simulink model "model15062023"  (R2021a)
settings: Solver=VariableStepAuto  StartTime=0.0  StopTime=10  FixedStep=1e-3  RelTol=1e-5
values from neighbouring files (symbols this model uses):
  I_max = 3*I_nom    (= 57.3875996726)    [LIM_parameters.m]
  I_min = 0.1*I_nom    (= 1.91291998909)    [LIM_parameters.m]
  I_nom = psi_ref/L_M_hat    (= 19.1291998909)    [LIM_parameters.m]
  ki_c = alpha_c*(R_hat+Ra )    [LIM_parameters.m]
  ki_s = alpha_s^2*m_hat/ psi_ref    [LIM_parameters.m]
  kp_c = alpha_c*L_sigma_hat    [LIM_parameters.m]
  kp_s = alpha_s*m_hat/ psi_ref    [LIM_parameters.m]
  L = 1    [LIM_parameters.m]
  L_alpha = (Ls+Lm)*(Lr+Lm) -Lm^2    (= 0.00742144)    [LIM_parameters.m]
  L_sigma_hat = L_sigma    (= 0.0268)    [LIM_parameters.m]
  Lm = 0.0416    [LIM_parameters.m]    (also in LIMvariables.m = 0.0376)
  Lr = 0.0416    [LIM_parameters.m]
  Ls = 0.0684    [LIM_parameters.m]
  m = 10    [LIM_parameters.m]    (also in LIMvariables.m)
  p = 4    [LIM_parameters.m]
  psi_ref = 1*250/(100*pi )    (= 0.795774715459)    [LIM_parameters.m]
  R_R_hat = Rr    (= 0.976)    [LIM_parameters.m]
  Ra = alpha_c*L_sigma_hat - R_hat    [LIM_parameters.m]
  Rr = 0.976    [LIM_parameters.m]
  Rs = 1.298    [LIM_parameters.m]
  tau = L/p    (= 0.25)    [LIM_parameters.m]    (also in LIMvariables.m = 0.066)
  V_sat = 415*sqrt(2/3)    [LIM_parameters.m]
  Vbase = 250    [LIM_parameters.m]
  wbase_fw = 50*2*pi    (= 314.159265359)    [LIM_parameters.m]
  zeta = (L_sigma_hat+L_M_hat)/L_sigma_hat    (= 2.55223880597)    [LIM_parameters.m]
libraries: simulink x5
settings Model: Creator=r.pitarque  LastModifiedBy=Asus

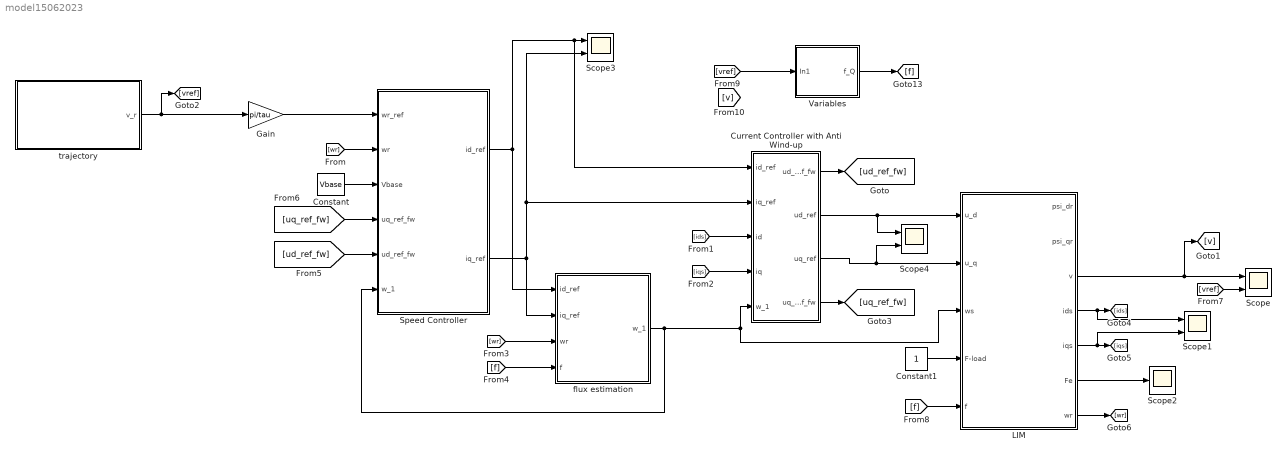
== system model15062023 ==
  Constant : Constant  Value=Vbase
  Constant1 : Constant
  Current Controller with Anti Wind-up : Subsystem
  Gain : Gain  Gain=pi/tau
  LIM : Subsystem
  Scope{,1,3..4} (4 alike) : Scope  NumInputPorts=2
  Scope2 : Scope
  Speed Controller : Subsystem
  Variables : Subsystem
  flux estimation : Subsystem
  trajectory : Subsystem
  wires:
  Current Controller with Anti Wind-up/1(ud_ref_fw) -> [ud_ref_fw]
  Current Controller with Anti Wind-up/2(ud_ref) -> Scope4/1, LIM/1(u_d)
  Current Controller with Anti Wind-up/3(uq_ref) -> Scope4/2, LIM/2(u_q)
  Current Controller with Anti Wind-up/4(uq_ref_fw) -> [uq_ref_fw]
  Speed Controller/1(id_ref) -> flux estimation/1(id_ref), Current Controller with Anti Wind-up/1(id_ref), Scope3/1
  LIM/4(ids) -> Scope1/1, [ids]
  LIM/5(iqs) -> Scope1/2, [iqs]
  LIM/7(wr) -> [wr]
  [wr] -> Speed Controller/2(wr)
  [ids] -> Current Controller with Anti Wind-up/3(id)
  [iqs] -> Current Controller with Anti Wind-up/4(iq)
  flux estimation/1(w_1) -> Speed Controller/6(w_1), Current Controller with Anti Wind-up/5(w_1), LIM/3(ws)
  [wr] -> flux estimation/3(wr)
  [f] -> flux estimation/4(f)
  Constant/1 -> Speed Controller/3(Vbase)
  [ud_ref_fw] -> Speed Controller/5(ud_ref_fw)
  [uq_ref_fw] -> Speed Controller/4(uq_ref_fw)
  trajectory/1(v_r) -> Gain/1, [vref]
  Gain/1 -> Speed Controller/1(wr_ref)
  LIM/3(v) -> [v], Scope/1
  [vref] -> Scope/2
  Variables/1(f_Q) -> [f]
  [f] -> LIM/5(f)
  LIM/6(Fe) -> Scope2/1
  Constant1/1 -> LIM/4(F-load)
  Speed Controller/2(iq_ref) -> flux estimation/2(iq_ref), Current Controller with Anti Wind-up/2(iq_ref), Scope3/2
  [vref] -> Variables/1(In1)

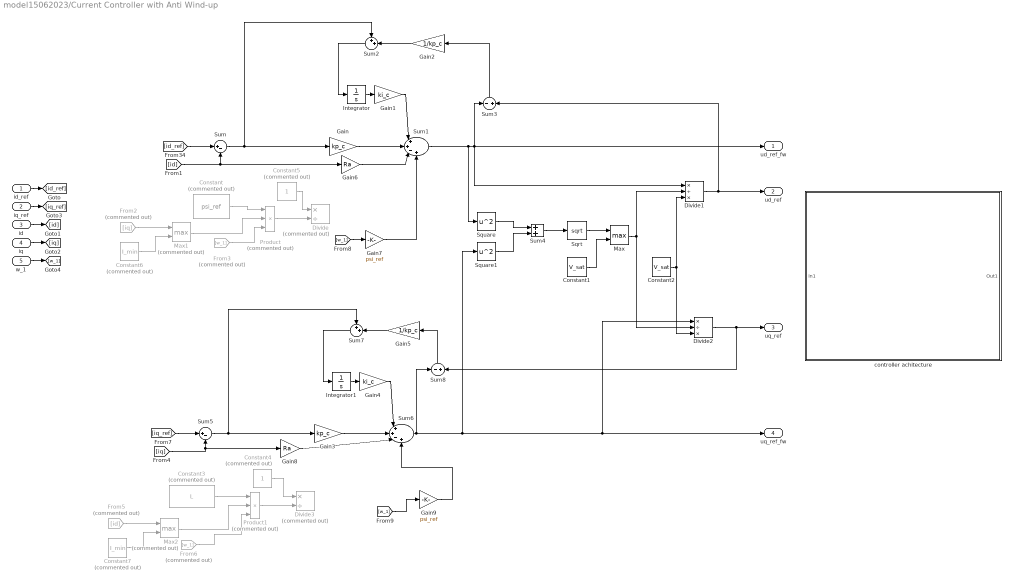
== system model15062023/Current Controller with Anti Wind-up ==
  id_ref : Inport
  iq_ref : Inport  Port=2
  id : Inport  Port=3
  iq : Inport  Port=4
  w_1 : Inport  Port=5
  Constant : Constant  Commented=on  Value=psi_ref
  Constant1 : Constant  Value=V_sat
  Constant2 : Constant  Value=V_sat
  Constant3 : Constant  Commented=on  Value=L
  Constant4 : Constant  Commented=on
  Constant5 : Constant  Commented=on
  Constant6 : Constant  Commented=on  Value=I_min
  Constant7 : Constant  Commented=on  Value=I_min
  Divide : Product  Commented=on  Inputs=*/
  Divide1 : Product  Inputs=*/*
  Divide2 : Product  Inputs=*/*
  Divide3 : Product  Commented=on  Inputs=*/
  From2 : From  Commented=on  GotoTag=iq
  From3 : From  Commented=on  GotoTag=w_1
  From5 : From  Commented=on  GotoTag=id
  From6 : From  Commented=on  GotoTag=w_1
  Gain : Gain  Gain=kp_c
  Gain1 : Gain  Gain=ki_c
  Gain2 : Gain  Gain=1/kp_c
  Gain3 : Gain  Gain=kp_c
  Gain4 : Gain  Gain=ki_c
  Gain5 : Gain  Gain=1/kp_c
  Gain6 : Gain  Gain=Ra
  Gain7 : Gain  Gain=psi_ref
  Gain8 : Gain  Gain=Ra
  Gain9 : Gain  Gain=psi_ref
  Integrator : Integrator
  Integrator1 : Integrator
  Max : MinMax  Function=max  Inputs=2
  Max1 : MinMax  Commented=on  Function=max  Inputs=2
  Max2 : MinMax  Commented=on  Function=max  Inputs=2
  Product : Product  Commented=on  Inputs=3
  Product1 : Product  Commented=on  Inputs=3
  Sqrt : Sqrt  SaturateOnIntegerOverflow=on
  Square : Math  Operator=square  SaturateOnIntegerOverflow=on
  Square1 : Math  Operator=square  SaturateOnIntegerOverflow=on
  Sum : Sum  Inputs=|+-
  Sum1 : Sum  Inputs=|++-+
  Sum2 : Sum  Inputs=++|
  Sum3 : Sum  Inputs=-+
  Sum4 : Sum
  Sum5 : Sum  Inputs=|+-
  Sum6 : Sum  Inputs=|++-+
  Sum7 : Sum  Inputs=++|
  Sum8 : Sum  Inputs=-+
  controller achitecture : Subsystem
      mask Display: image('C:\Users\Asus\Desktop\cc.png'); % Use "Edit Image" on toolstrip to change.
  ud_ref_fw : Outport
  ud_ref : Outport  Port=2
  uq_ref : Outport  Port=3
  uq_ref_fw : Outport  Port=4
  wires:
  Square/1 -> Sum4/1
  Constant1/1 -> Max/2
  Sum6/1 -> Sum8/1, uq_ref_fw/1, Divide2/1, Square1/1
  Max/1 -> Divide2/2, Divide1/2
  Sum1/1 -> ud_ref_fw/1, Sum3/1, Divide1/1, Square/1
  Constant3/1 -> Product1/1
  Square1/1 -> Sum4/2
  Constant2/1 -> Divide1/3, Divide2/3
  Gain1/1 -> Sum1/1
  Divide2/1 -> uq_ref/1, Sum8/2
  Sqrt/1 -> Max/1
  Sum/1 -> Gain/1, Sum2/1
  Sum4/1 -> Sqrt/1
  Product/1 -> Divide/2
  Gain2/1 -> Sum2/2
  Divide1/1 -> ud_ref/1, Sum3/2
  Integrator/1 -> Gain1/1
  Sum5/1 -> Gain3/1, Sum7/1
  Constant/1 -> Product/1
  Gain/1 -> Sum1/2
  Integrator1/1 -> Gain4/1
  Gain4/1 -> Sum6/1
  Sum3/1 -> Gain2/1
  Sum7/1 -> Integrator1/1
  Gain3/1 -> Sum6/2
  Product1/1 -> Divide3/2
  Sum8/1 -> Gain5/1
  Sum2/1 -> Integrator/1
  [id_ref] -> Sum/1
  [id] -> Gain6/1, Sum/2
  From6/1 -> Product1/3
  [iq_ref] -> Sum5/1
  [iq] -> Gain8/1, Sum5/2
  From2/1 -> Max1/1
  From3/1 -> Product/3
  id/1 -> [id]
  iq/1 -> [iq]
  w_1/1 -> [w_1]
  iq_ref/1 -> [iq_ref]
  id_ref/1 -> [id_ref]
  Gain5/1 -> Sum7/2
  Constant4/1 -> Divide3/1
  Constant5/1 -> Divide/1
  Constant6/1 -> Max1/2
  Max1/1 -> Product/2
  Constant7/1 -> Max2/2
  From5/1 -> Max2/1
  Max2/1 -> Product1/2
  Gain6/1 -> Sum1/3
  [w_1] -> Gain7/1
  Gain7/1 -> Sum1/4
  Gain8/1 -> Sum6/3
  [w_1] -> Gain9/1
  Gain9/1 -> Sum6/4

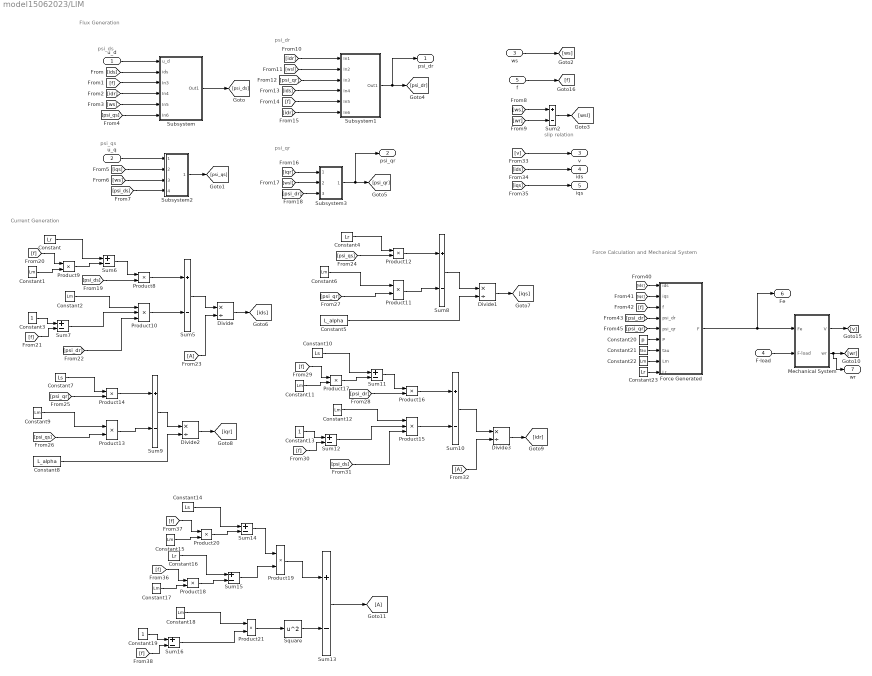
== system model15062023/LIM ==
  note: Force Calculation and Mechanical System
  note: Current Generation
  note: Flux Generation
  note: psi_qr
  note: psi_dr
  note: psi_qs
  note: psi_ds
  note: slip relation
  u_d : Inport
  u_q : Inport  Port=2
  ws : Inport  Port=3
  F-load : Inport  Port=4
  f : Inport  Port=5
  Constant{,4,16,23} (4 alike) : Constant  Value=Lr
  Constant{1..2,6,9,11..12,15,17..18,22} (10 alike) : Constant  Value=Lm
  Constant10 : Constant  Value=Ls
  Constant13 : Constant
  Constant14 : Constant  Value=Ls
  Constant19 : Constant
  Constant20 : Constant  Value=p
  Constant21 : Constant  Value=tau
  Constant3 : Constant
  Constant5 : Constant  Value=L_alpha
  Constant7 : Constant  Value=Ls
  Constant8 : Constant  Value=L_alpha
  Divide{,1..3} (4 alike) : Product  Inputs=*/
  Force Generated : MATLAB Function  TreatAsAtomicUnit=on
  Mechanical System : Subsystem
  Product10 : Product  Inputs=3
  Product{8..9,11..14,16..21} (12 alike) : Product
  Product15 : Product  Inputs=3
  Square : Math  Operator=square  SaturateOnIntegerOverflow=on
  Subsystem : Subsystem
  Subsystem1 : Subsystem
  Subsystem2 : Subsystem
  Subsystem3 : Subsystem
  Sum{2,5..16} (13 alike) : Sum  Inputs=+-
  psi_dr : Outport
  psi_qr : Outport  Port=2
  v : Outport  Port=3
  ids : Outport  Port=4
  iqs : Outport  Port=5
  Fe : Outport  Port=6
  wr : Outport  Port=7
  wires:
  [f] -> Sum16/2
  [psi_qs] -> Product12/2
  Constant3/1 -> Sum7/1
  Constant16/1 -> Sum15/1
  [v] -> v/1
  Divide1/1 -> [iqs]
  Constant19/1 -> Sum16/1
  [f] -> Sum7/2
  [ws] -> Sum2/1
  Sum5/1 -> Divide/1
  Constant12/1 -> Product15/1
  Sum6/1 -> Product8/1
  [psi_dr] -> Subsystem3/3(In3)
  Divide/1 -> [ids]
  [psi_qr] -> Force Generated/5(psi_qr)
  [A] -> Divide/2
  Sum13/1 -> [A]
  [f] -> Product17/1
  Product10/1 -> Sum5/2
  Force Generated/1(F) -> Fe/1, Mechanical System/1(Fe)
  [psi_ds] -> Product15/3
  [psi_qr] -> Product11/2
  Constant8/1 -> Divide2/2
  Divide2/1 -> [iqr]
  Sum7/1 -> Product10/2
  Constant14/1 -> Sum14/1
  F-load/1 -> Mechanical System/2(F-load)
  [iqs] -> iqs/1
  Constant9/1 -> Product13/1
  Sum2/1 -> [wsl]
  Sum9/1 -> Divide2/1
  [f] -> Product9/1
  Sum8/1 -> Divide1/1
  Product13/1 -> Sum9/2
  Constant1/1 -> Product9/2
  [psi_qr] -> Product14/2
  Constant7/1 -> Product14/1
  Square/1 -> Sum13/2
  [wsl] -> Subsystem1/2(In2)
  Product14/1 -> Sum9/1
  [idr] -> Subsystem1/1(In1)
  [ids] -> Force Generated/1(ids)
  [psi_qs] -> Product13/2
  [idr] -> Subsystem1/6(In6)
  [psi_qr] -> Subsystem1/3(In3)
  Product12/1 -> Sum8/1
  Mechanical System/2(wr) -> wr/1, [wr]
  Subsystem1/1(Out1) -> psi_dr/1, [psi_dr]
  [f] -> Product20/1
  Product21/1 -> Square/1
  Product11/1 -> Sum8/2
  Sum15/1 -> Product19/2
  Product9/1 -> Sum6/2
  Subsystem/1(Out1) -> [psi_ds]
  Subsystem3/1(Out1) -> psi_qr/1, [psi_qr]
  Constant2/1 -> Product10/1
  [f] -> Subsystem1/5(In5)
  ws/1 -> [ws]
  [wr] -> Sum2/2
  [psi_dr] -> Product10/3
  [psi_dr] -> Force Generated/4(psi_dr)
  Constant18/1 -> Product21/1
  [ws] -> Subsystem2/3(In3)
  Constant4/1 -> Product12/1
  Constant/1 -> Sum6/1
  Constant6/1 -> Product11/1
  Constant21/1 -> Force Generated/7(tau)
  Product8/1 -> Sum5/1
  [f] -> Product18/1
  Constant17/1 -> Product18/2
  Product18/1 -> Sum15/2
  [psi_ds] -> Product8/2
  Constant5/1 -> Divide1/2
  Sum16/1 -> Product21/2
  [psi_dr] -> Product16/2
  Product16/1 -> Sum10/1
  Sum12/1 -> Product15/2
  Constant11/1 -> Product17/2
  [f] -> Sum12/2
  Constant10/1 -> Sum11/1
  Product17/1 -> Sum11/2
  Product15/1 -> Sum10/2
  [A] -> Divide3/2
  Constant23/1 -> Force Generated/9(Lr)
  Divide3/1 -> [idr]
  Constant13/1 -> Sum12/1
  Sum11/1 -> Product16/1
  Sum10/1 -> Divide3/1
  [ids] -> ids/1
  Product20/1 -> Sum14/2
  Constant15/1 -> Product20/2
  Sum14/1 -> Product19/1
  Product19/1 -> Sum13/1
  Mechanical System/1(V) -> [v]
  [f] -> Force Generated/3(f)
  Constant20/1 -> Force Generated/6(P)
  [ws] -> Subsystem/5(In5)
  [psi_qs] -> Subsystem/6(In6)
  u_d/1 -> Subsystem/1(u_d)
  [idr] -> Subsystem/4(In4)
  [f] -> Subsystem/3(In3)
  [ids] -> Subsystem/2(ids)
  [iqs] -> Force Generated/2(iqs)
  [ids] -> Subsystem1/4(In4)
  [iqr] -> Subsystem3/1(In1)
  [wsl] -> Subsystem3/2(In2)
  [psi_ds] -> Subsystem2/4(In4)
  Subsystem2/1(Out1) -> [psi_qs]
  [iqs] -> Subsystem2/2(In2)
  u_q/1 -> Subsystem2/1(In1)
  Constant22/1 -> Force Generated/8(Lm)
  f/1 -> [f]

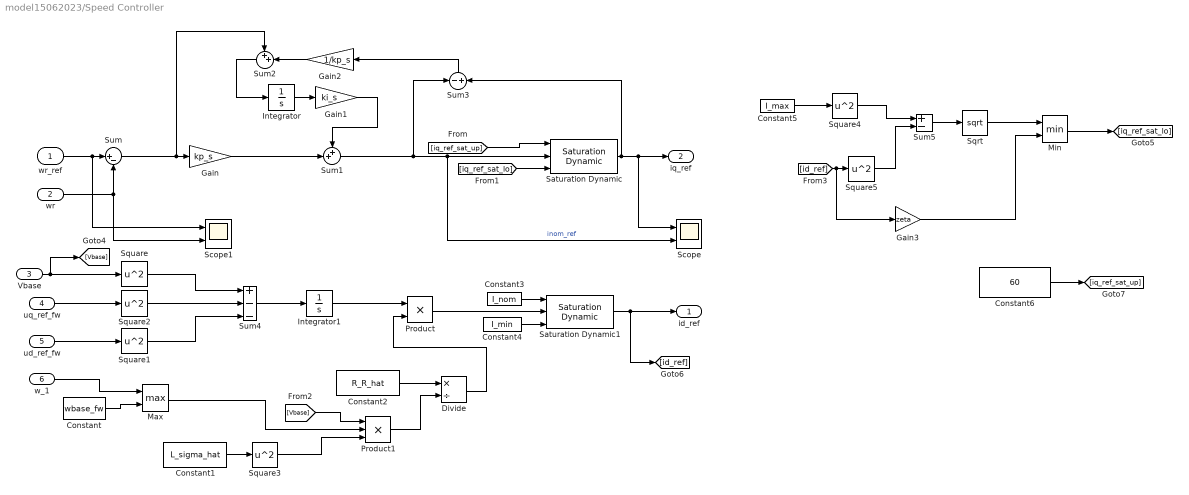
== system model15062023/Speed Controller ==
  wr_ref : Inport
  wr : Inport  Port=2
  Vbase : Inport  Port=3
  uq_ref_fw : Inport  Port=4
  ud_ref_fw : Inport  Port=5
  w_1 : Inport  Port=6
  Constant : Constant  Value=wbase_fw
  Constant1 : Constant  Value=L_sigma_hat
  Constant2 : Constant  Value=R_R_hat
  Constant3 : Constant  Value=I_nom
  Constant4 : Constant  Value=I_min
  Constant5 : Constant  Value=I_max
  Constant6 : Constant  Value=60
  Divide : Product  Inputs=*/
  Gain : Gain  Gain=kp_s
  Gain1 : Gain  Gain=ki_s
  Gain2 : Gain  Gain=1/kp_s
  Gain3 : Gain  Gain=zeta
  Integrator : Integrator
  Integrator1 : Integrator
  Max : MinMax  Function=max  Inputs=2
  Min : MinMax  Inputs=2
  Product : Product
  Product1 : Product  Inputs=3
  Saturation Dynamic : simulink/Discontinuities/Saturation Dynamic  OutMin=[]  OutMax=[]  OutDataTypeStr=Inherit: Same as second input  OutDataType=fixdt(1, 16)  OutScaling=2^-10  DoSatur=off
  Saturation Dynamic1 : simulink/Discontinuities/Saturation Dynamic  OutMin=[]  OutMax=[]  OutDataTypeStr=Inherit: Same as second input  OutDataType=fixdt(1, 16)  OutScaling=2^-10  DoSatur=off
  Scope : Scope  NumInputPorts=2
  Scope1 : Scope  NumInputPorts=2
  Sqrt : Sqrt  SaturateOnIntegerOverflow=on
  Square{,1..5} (6 alike) : Math  Operator=square  SaturateOnIntegerOverflow=on
  Sum : Sum  Inputs=|+-
  Sum1 : Sum  Inputs=++|
  Sum2 : Sum  Inputs=++|
  Sum3 : Sum  Inputs=-+
  Sum4 : Sum  Inputs=+--
  Sum5 : Sum  Inputs=+-
  id_ref : Outport
  iq_ref : Outport  Port=2
  wires:
  Constant2/1 -> Divide/1
  Integrator1/1 -> Product/1
  Gain2/1 -> Sum2/2
  Square1/1 -> Sum4/3
  Min/1 -> [iq_ref_sat_lo]
  Constant5/1 -> Square4/1
  Vbase/1 -> [Vbase], Square/1
  Constant4/1 -> Saturation Dynamic1/3
  Gain3/1 -> Min/2
  Sum/1 -> Sum2/1, Gain/1
  Product1/1 -> Divide/2
  Constant3/1 -> Saturation Dynamic1/1
  [Vbase] -> Product1/1
  Max/1 -> Product1/2
  Square5/1 -> Sum5/2
  Saturation Dynamic1/1 -> id_ref/1, [id_ref]
  Constant/1 -> Max/2
  [iq_ref_sat_lo] -> Saturation Dynamic/3
  [id_ref] -> Gain3/1, Square5/1
  Gain/1 -> Sum1/2
  uq_ref_fw/1 -> Square2/1
  Sum5/1 -> Sqrt/1
  Constant1/1 -> Square3/1
  Sum4/1 -> Integrator1/1
  Sum3/1 -> Gain2/1
  Product/1 -> Saturation Dynamic1/2
  Square2/1 -> Sum4/2
  [iq_ref_sat_up] -> Saturation Dynamic/1
  ud_ref_fw/1 -> Square1/1
  Divide/1 -> Product/2
  Sqrt/1 -> Min/1
  Square4/1 -> Sum5/1
  Sum2/1 -> Integrator/1
  wr/1 -> Scope1/2, Sum/2
  Square/1 -> Sum4/1
  Sum1/1 -> Scope/2, Saturation Dynamic/2, Sum3/1  "inom_ref"
  w_1/1 -> Max/1
  Constant6/1 -> [iq_ref_sat_up]
  Integrator/1 -> Gain1/1
  Square3/1 -> Product1/3
  Saturation Dynamic/1 -> Scope/1, iq_ref/1, Sum3/2
  Gain1/1 -> Sum1/1
  wr_ref/1 -> Scope1/1, Sum/1

== system model15062023/Variables ==
  In1 : Inport
  Gain : Gain  Gain=L*Rr/Lr
  Subsystem5 : Subsystem  Commented=on
  f(Q) : MATLAB Function  TreatAsAtomicUnit=on
  f_Q : Outport
  wires:
  Gain/1 -> f(Q)/1(u)  "Q"
  f(Q)/1(y) -> f_Q/1, Subsystem5/1(f_q)  "F_Q"
  Subsystem5/1(Lsigma) -> ?
  In1/1 -> Gain/1

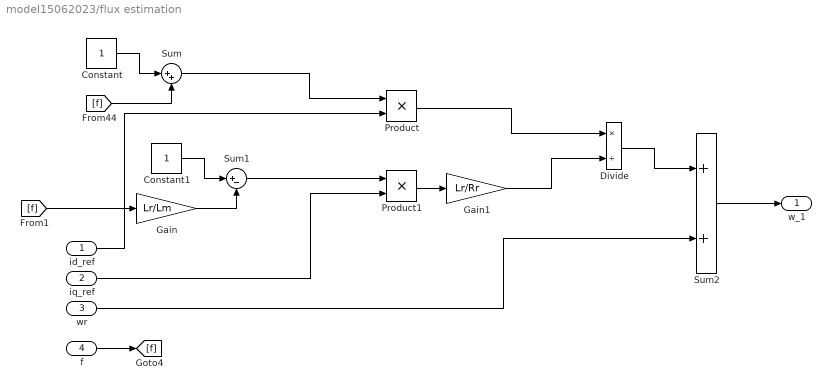
== system model15062023/flux estimation ==
  id_ref : Inport
  iq_ref : Inport  Port=2
  wr : Inport  Port=3
  f : Inport  Port=4
  Constant : Constant
  Constant1 : Constant
  Divide : Product  Inputs=*/
  Gain : Gain  Gain=Lr/Lm
  Gain1 : Gain  Gain=Lr/Rr
  Product : Product
  Product1 : Product
  Sum : Sum  Inputs=|++
  Sum1 : Sum  Inputs=|+-
  Sum2 : Sum
  w_1 : Outport
  wires:
  Sum1/1 -> Product1/1
  Divide/1 -> Sum2/1
  wr/1 -> Sum2/2
  Product/1 -> Divide/1
  Constant/1 -> Sum/1
  Gain/1 -> Sum1/2
  id_ref/1 -> Product/2
  Gain1/1 -> Divide/2
  [f] -> Sum/2
  Product1/1 -> Gain1/1
  Sum/1 -> Product/1
  Constant1/1 -> Sum1/1
  [f] -> Gain/1
  iq_ref/1 -> Product1/2
  f/1 -> [f]
  Sum2/1 -> w_1/1

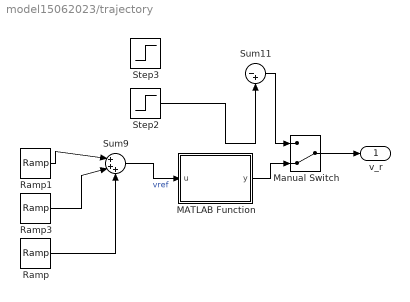
== system model15062023/trajectory ==
  MATLAB Function : MATLAB Function  TreatAsAtomicUnit=on
  Manual Switch : ManualSwitch  CurrentSetting=0
  Ramp : simulink/Sources/Ramp  slope=-6.5  start=5.28  InitialOutput=0
  Ramp1 : simulink/Sources/Ramp  slope=4.12  start=0  InitialOutput=0.1
  Ramp3 : simulink/Sources/Ramp  slope=-4.12  start=5.28  InitialOutput=0.1
  Step2 : Step  Time=0  Before=0.1  SampleTime=0
  Step3 : Step  Time=4  Before=20  After=0.1  SampleTime=0
  Sum11 : Sum  Inputs=|-+
  Sum9 : Sum  Inputs=|+++
  v_r : Outport
  wires:
  MATLAB Function/1(y) -> Manual Switch/2
  Sum11/1 -> Manual Switch/1
  Ramp3/1 -> Sum9/2
  Step2/1 -> Sum11/2
  Ramp/1 -> Sum9/3
  Ramp1/1 -> Sum9/1
  Manual Switch/1 -> v_r/1
  Sum9/1 -> MATLAB Function/1(u)  "vref"

== system model15062023/Current Controller with Anti Wind-up/controller achitecture ==
  In1 : Inport
  Out1 : Outport
  wires:
  In1/1 -> Out1/1

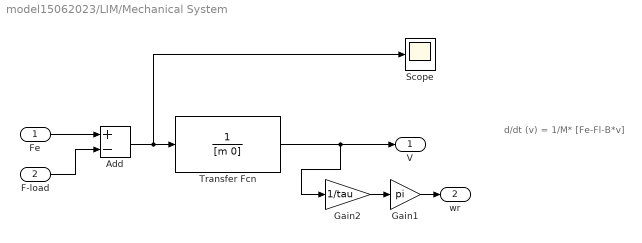
== system model15062023/LIM/Mechanical System ==
  note: d/dt (v) = 1/M* [Fe-Fl-B*v]
  Fe : Inport
  F-load : Inport  Port=2
  Add : Sum  Inputs=+-
  Gain1 : Gain  Gain=pi
  Gain2 : Gain  Gain=1/tau
  Scope : Scope
  Transfer Fcn : TransferFcn  Denominator=[m 0]
  V : Outport
  wr : Outport  Port=2
  wires:
  Fe/1 -> Add/1
  F-load/1 -> Add/2
  Add/1 -> Scope/1, Transfer Fcn/1
  Gain2/1 -> Gain1/1
  Gain1/1 -> wr/1
  Transfer Fcn/1 -> Gain2/1, V/1

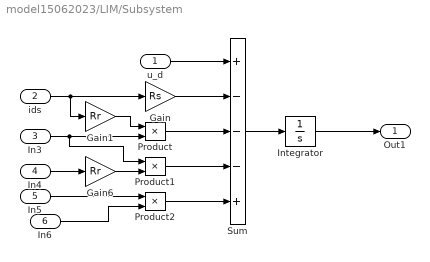
== system model15062023/LIM/Subsystem ==
  u_d : Inport
  ids : Inport  Port=2
  In3 : Inport  Port=3
  In4 : Inport  Port=4
  In5 : Inport  Port=5
  In6 : Inport  Port=6
  Gain : Gain  Gain=Rs
  Gain1 : Gain  Gain=Rr
  Gain6 : Gain  Gain=Rr
  Integrator : Integrator
  Product : Product
  Product1 : Product
  Product2 : Product
  Sum : Sum  Inputs=+---+
  Out1 : Outport
  wires:
  Gain1/1 -> Product/1
  Product/1 -> Sum/3
  ids/1 -> Gain1/1, Gain/1
  Product2/1 -> Sum/5
  Gain/1 -> Sum/2
  In3/1 -> Product1/1, Product/2
  u_d/1 -> Sum/1
  Product1/1 -> Sum/4
  Sum/1 -> Integrator/1
  Gain6/1 -> Product1/2
  In5/1 -> Product2/1
  In6/1 -> Product2/2
  In4/1 -> Gain6/1
  Integrator/1 -> Out1/1

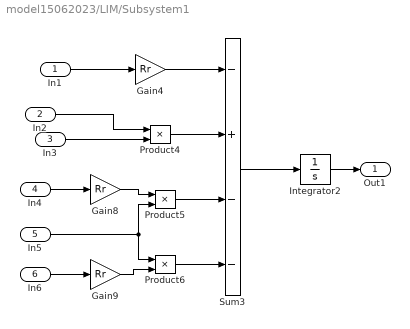
== system model15062023/LIM/Subsystem1 ==
  In1 : Inport
  In2 : Inport  Port=2
  In3 : Inport  Port=3
  In4 : Inport  Port=4
  In5 : Inport  Port=5
  In6 : Inport  Port=6
  Gain4 : Gain  Gain=Rr
  Gain8 : Gain  Gain=Rr
  Gain9 : Gain  Gain=Rr
  Integrator2 : Integrator
  Product4 : Product
  Product5 : Product
  Product6 : Product
  Sum3 : Sum  Inputs=-+--
  Out1 : Outport
  wires:
  Gain9/1 -> Product6/2
  Product4/1 -> Sum3/2
  Product6/1 -> Sum3/4
  Integrator2/1 -> Out1/1
  Gain8/1 -> Product5/1
  In5/1 -> Product6/1, Product5/2
  Sum3/1 -> Integrator2/1
  Product5/1 -> Sum3/3
  Gain4/1 -> Sum3/1
  In1/1 -> Gain4/1
  In3/1 -> Product4/2
  In2/1 -> Product4/1
  In4/1 -> Gain8/1
  In6/1 -> Gain9/1

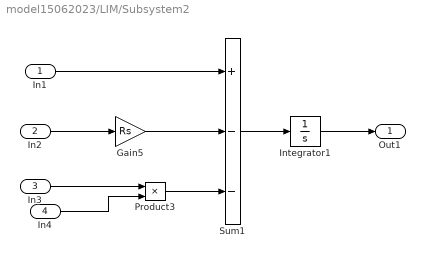
== system model15062023/LIM/Subsystem2 ==
  In1 : Inport
  In2 : Inport  Port=2
  In3 : Inport  Port=3
  In4 : Inport  Port=4
  Gain5 : Gain  Gain=Rs
  Integrator1 : Integrator
  Product3 : Product
  Sum1 : Sum  Inputs=+--
  Out1 : Outport
  wires:
  Integrator1/1 -> Out1/1
  Gain5/1 -> Sum1/2
  In3/1 -> Product3/1
  In1/1 -> Sum1/1
  Product3/1 -> Sum1/3
  Sum1/1 -> Integrator1/1
  In2/1 -> Gain5/1
  In4/1 -> Product3/2

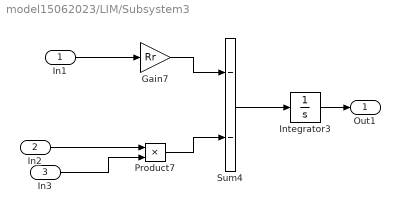
== system model15062023/LIM/Subsystem3 ==
  In1 : Inport
  In2 : Inport  Port=2
  In3 : Inport  Port=3
  Gain7 : Gain  Gain=Rr
  Integrator3 : Integrator
  Product7 : Product
  Sum4 : Sum  Inputs=--
  Out1 : Outport
  wires:
  In2/1 -> Product7/1
  Product7/1 -> Sum4/2
  Gain7/1 -> Sum4/1
  Sum4/1 -> Integrator3/1
  In1/1 -> Gain7/1
  Integrator3/1 -> Out1/1
  In3/1 -> Product7/2

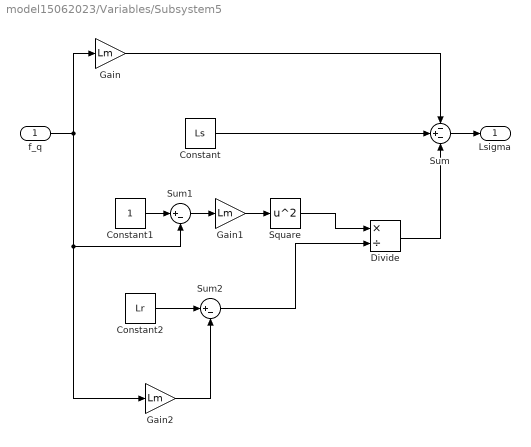
== system model15062023/Variables/Subsystem5 ==
  f_q : Inport
  Constant : Constant  Value=Ls
  Constant1 : Constant
  Constant2 : Constant  Value=Lr
  Divide : Product  Inputs=*/
  Gain : Gain  Gain=Lm
  Gain1 : Gain  Gain=Lm
  Gain2 : Gain  Gain=Lm
  Square : Math  Operator=square  SaturateOnIntegerOverflow=on
  Sum : Sum  Inputs=-+-
  Sum1 : Sum  Inputs=|+-
  Sum2 : Sum  Inputs=|+-
  Lsigma : Outport
  wires:
  Constant/1 -> Sum/2
  f_q/1 -> Sum1/2, Gain2/1, Gain/1
  Gain/1 -> Sum/1
  Sum/1 -> Lsigma/1
  Constant1/1 -> Sum1/1
  Sum1/1 -> Gain1/1
  Gain1/1 -> Square/1
  Square/1 -> Divide/1
  Constant2/1 -> Sum2/1
  Gain2/1 -> Sum2/2
  Sum2/1 -> Divide/2
  Divide/1 -> Sum/3

== matlab function model15062023/LIM/Force Generated ==
  data: ids input; iqs input; f input; psi_dr input; psi_qr input; F output; P input; tau input; Lm input; Lr input
function F = fcn(ids,iqs,f,psi_dr,psi_qr,P,tau,Lm,Lr)

F = ((3*P*pi)/2*tau)*(Lm*(1-f)/(Lr-Lm*f))*(psi_dr*iqs-psi_qr*ids);

== matlab function model15062023/Variables/f(Q) ==
  data: u input; y output
function y = fcn(u)

y = (1-exp(-u))/u;

== matlab function model15062023/trajectory/MATLAB Function ==
  data: u input; y output
function y = fcn(u)

if u ~= 0
    y = u;
else
    y = 1;
end
